simulink model "Chua_normal"  (R2020a)
settings: Solver=VariableStepAuto  StartTime=0.0  StopTime=1000  RelTol=1e-3
settings Model: PacingRate=1.100000  Creator=RaviM  LastModifiedBy=RaviM

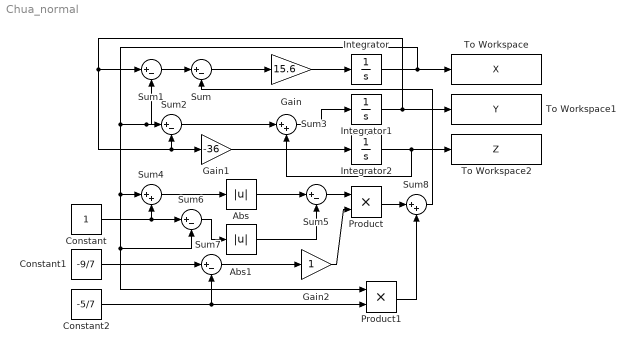
== system Chua_normal ==
  Abs : Abs
  Abs1 : Abs
  Constant : Constant
  Constant1 : Constant  Value=-9/7
  Constant2 : Constant  Value=-5/7
  Gain : Gain  Gain=15.6
  Gain1 : Gain  Gain=-36
  Gain2 : Gain
  Integrator : Integrator  InitialCondition=0.1
  Integrator1 : Integrator  InitialCondition=0.1
  Integrator2 : Integrator  InitialCondition=0.1
  Product : Product
  Product1 : Product
  Sum{,1..2,5..7} (6 alike) : Sum  Inputs=|+-
  Sum3 : Sum  Inputs=|++
  Sum4 : Sum  Inputs=|++
  Sum8 : Sum  Inputs=|++
  To Workspace : ToWorkspace  VariableName=X  SaveFormat=Timeseries  SampleTime=-1
  To Workspace1 : ToWorkspace  VariableName=Y  SaveFormat=Timeseries  SampleTime=-1
  To Workspace2 : ToWorkspace  VariableName=Z  SaveFormat=Timeseries  SampleTime=-1
  wires:
  Constant2/1 -> Product1/2, Sum7/2
  Constant1/1 -> Sum7/1
  Sum7/1 -> Gain2/1
  Gain2/1 -> Product/2
  Product1/1 -> Sum8/2
  Product/1 -> Sum8/1
  Sum6/1 -> Abs1/1
  Sum4/1 -> Abs/1
  Abs/1 -> Sum5/1
  Abs1/1 -> Sum5/2
  Constant/1 -> Sum6/1, Sum4/2
  Sum8/1 -> Sum/2
  Sum1/1 -> Sum/1
  Sum/1 -> Gain/1
  Gain/1 -> Integrator/1
  Sum3/1 -> Integrator1/1
  Sum2/1 -> Sum3/1
  Integrator1/1 -> Gain1/1, Sum2/2, Sum1/1, To Workspace1/1
  Integrator2/1 -> Sum3/2, To Workspace2/1
  Integrator/1 -> Product1/1, Sum6/2, Sum4/1, Sum1/2, Sum2/1, To Workspace/1
  Gain1/1 -> Integrator2/1
  Sum5/1 -> Product/1
